simulink model "SimulateROSBag"  (R2020b)
settings: Solver=VariableStepAuto  StartTime=0.0  StopTime=80  RelTol=1e-3
PreLoadFcn:
  | load('turtleBotMazeMap.mat')
model workspace (MAT data in the model file):
  Logfile_Data_Object = robotics.ros.BagSelection
  Logfile_Data_Object.FilePath = 'C:\Users\josea\OneDrive - MathWorks\Desktop\RoboticsArena\Navigation_Series\MATLAB_Files\CreatingMaps\Data\ROSBag_turtleBotMaze.bag'
  Logfile_Data_Object.StartTime = 1574.403
  Logfile_Data_Object.EndTime = 1757.346
  Logfile_Data_Object.NumMessages = 6404
  Logfile_Data_Object.AvailableTopics = table
  Logfile_Data_Object.AvailableTopics.data{1} = [5489; 915]
  Logfile_Data_Object.AvailableTopics.data{2} = categorical
  Logfile_Data_Object.AvailableTopics.data{2}.categoryNames = {'nav_msgs/Odometry'; 'sensor_msgs/LaserScan'}
  Logfile_Data_Object.AvailableTopics.data{2}.codes = [1; 2]
  Logfile_Data_Object.AvailableTopics.data{3}{1} = '  uint32 Seq
    |   Time Stamp
    |   char FrameId
    | char ChildFrameId
    | geometry_msgs/PoseWithCovariance Pose
    |   geometry_msgs/Pose Pose
    |     geometry_msgs/Point Position
    |       double X
    |       double Y
    |       double Z
    |     geometry_msgs/Quaternion Orientation
    |       double X
    |       double Y
    |       double Z
    |       double W
    |   double[36] Covariance
    | geometry_msgs/TwistWithCovariance Twist
    |   geometry_msgs/Twist Twist
    |     geometry_msgs/Vector3 Linear
    |       double X
    |       double Y
    |       double Z
    |     geometry_msgs/Vector3 Angular
    |       double X
    |       double Y
    |       double Z
    |   double[36] Covariance
    | '
  Logfile_Data_Object.AvailableTopics.data{3}{2} = '  uint32 Seq
    |   Time Stamp
    |   char FrameId
    | single AngleMin
    | single AngleMax
    | single AngleIncrement
    | single TimeIncrement
    | single ScanTime
    | single RangeMin
    | single RangeMax
    | single[] Ranges
    | single[] Intensities
    | '
  Logfile_Data_Object.AvailableTopics.ndims = 2
  Logfile_Data_Object.AvailableTopics.nrows = 2
  Logfile_Data_Object.AvailableTopics.rownames = {'/odom'; '/scan'}
  Logfile_Data_Object.AvailableTopics.nvars = 3
  Logfile_Data_Object.AvailableTopics.varnames = {'NumMessages', 'MessageType', 'MessageDefinition'}
  Logfile_Data_Object.AvailableTopics.props.useVariableNamesOriginal = 0
  Logfile_Data_Object.AvailableTopics.props.useDimensionNamesOriginal = 0
  Logfile_Data_Object.AvailableTopics.props.CustomProps = struct()
  Logfile_Data_Object.AvailableTopics.props.VariableCustomProps = struct()
  Logfile_Data_Object.AvailableTopics.props.versionSavedFrom = 4
  Logfile_Data_Object.AvailableTopics.props.minCompatibleVersion = 1
  Logfile_Data_Object.AvailableTopics.props.incompatibilityMsg = ''
  Logfile_Data_Object.AvailableTopics.props.VersionSavedFrom = 4
  Logfile_Data_Object.AvailableTopics.props.Description = ''
  Logfile_Data_Object.AvailableTopics.props.VariableNamesOriginal = {}
  Logfile_Data_Object.AvailableTopics.props.DimensionNames = {'Row', 'Variables'}
  Logfile_Data_Object.AvailableTopics.props.DimensionNamesOriginal = {}
  Logfile_Data_Object.AvailableTopics.props.UserData = []
  Logfile_Data_Object.AvailableTopics.props.VariableDescriptions = {}
  Logfile_Data_Object.AvailableTopics.props.VariableUnits = {}
  Logfile_Data_Object.AvailableTopics.props.VariableContinuity = {}
  Logfile_Data_Object.MessageList = table
  Logfile_Data_Object.MessageList.data{1} = [1574.403 1574.437 1574.469 1574.502 1574.503 1574.537 1574.57 1574.603 1574.637 1574.67 1574.702 1574.704 ... (6404 elements, 6404x1)]
  Logfile_Data_Object.MessageList.data{2} = categorical
  Logfile_Data_Object.MessageList.data{2}.categoryNames = {'/odom'; '/scan'}
  Logfile_Data_Object.MessageList.data{2}.codes = [1 1 1 2 1 1 1 1 1 1 1 2 ... (6404 elements, 6404x1)]
  Logfile_Data_Object.MessageList.data{3} = categorical
  Logfile_Data_Object.MessageList.data{3}.categoryNames = {'nav_msgs/Odometry'; 'sensor_msgs/LaserScan'}
  Logfile_Data_Object.MessageList.data{3}.codes = [1 1 1 2 1 1 1 1 1 1 1 2 ... (6404 elements, 6404x1)]
  Logfile_Data_Object.MessageList.data{4} = [7630 8394 9158 12284 15271 16035 16799 17563 18327 19091 19855 20619 ... (6404 elements, 6404x1)]
  Logfile_Data_Object.MessageList.ndims = 2
  Logfile_Data_Object.MessageList.nrows = 6404
  Logfile_Data_Object.MessageList.nvars = 4
  Logfile_Data_Object.MessageList.varnames = {'Time', 'Topic', 'MessageType', 'FileOffset'}
  Logfile_Data_Object.MessageList.props.useVariableNamesOriginal = 0
  Logfile_Data_Object.MessageList.props.useDimensionNamesOriginal = 0
  Logfile_Data_Object.MessageList.props.CustomProps = struct()
  Logfile_Data_Object.MessageList.props.VariableCustomProps = struct()
  Logfile_Data_Object.MessageList.props.versionSavedFrom = 4
  Logfile_Data_Object.MessageList.props.minCompatibleVersion = 1
  Logfile_Data_Object.MessageList.props.incompatibilityMsg = ''
  Logfile_Data_Object.MessageList.props.VersionSavedFrom = 4
  Logfile_Data_Object.MessageList.props.Description = ''
  Logfile_Data_Object.MessageList.props.VariableNamesOriginal = {}
  Logfile_Data_Object.MessageList.props.DimensionNames = {'Row', 'Variables'}
  Logfile_Data_Object.MessageList.props.DimensionNamesOriginal = {}
  Logfile_Data_Object.MessageList.props.UserData = []
  Logfile_Data_Object.MessageList.props.VariableDescriptions = {}
  Logfile_Data_Object.MessageList.props.VariableUnits = {}
  Logfile_Data_Object.MessageList.props.VariableContinuity = {}
  Logfile_Data_Object.TopicTypeMap = containers.Map
  Logfile_Data_Object.TopicTypeMap.serialization.keys = {'/odom', '/scan'}
  Logfile_Data_Object.TopicTypeMap.serialization.values = {'nav_msgs/Odometry', 'sensor_msgs/LaserScan'}
  Logfile_Data_Object.TopicTypeMap.serialization.uniformity = 1
  Logfile_Data_Object.TopicTypeMap.serialization.keyType = 'char'
  Logfile_Data_Object.TopicTypeMap.serialization.valueType = 'char'
  Logfile_Data_Object.TopicDefinitionMap = containers.Map
  Logfile_Data_Object.TopicDefinitionMap.serialization.keys = {'/odom', '/scan'}
  Logfile_Data_Object.TopicDefinitionMap.serialization.values{1} = '  uint32 Seq
    |   Time Stamp
    |   char FrameId
    | char ChildFrameId
    | geometry_msgs/PoseWithCovariance Pose
    |   geometry_msgs/Pose Pose
    |     geometry_msgs/Point Position
    |       double X
    |       double Y
    |       double Z
    |     geometry_msgs/Quaternion Orientation
    |       double X
    |       double Y
    |       double Z
    |       double W
    |   double[36] Covariance
    | geometry_msgs/TwistWithCovariance Twist
    |   geometry_msgs/Twist Twist
    |     geometry_msgs/Vector3 Linear
    |       double X
    |       double Y
    |       double Z
    |     geometry_msgs/Vector3 Angular
    |       double X
    |       double Y
    |       double Z
    |   double[36] Covariance
    | '
  Logfile_Data_Object.TopicDefinitionMap.serialization.values{2} = '  uint32 Seq
    |   Time Stamp
    |   char FrameId
    | single AngleMin
    | single AngleMax
    | single AngleIncrement
    | single TimeIncrement
    | single ScanTime
    | single RangeMin
    | single RangeMax
    | single[] Ranges
    | single[] Intensities
    | '
  Logfile_Data_Object.TopicDefinitionMap.serialization.uniformity = 1
  Logfile_Data_Object.TopicDefinitionMap.serialization.keyType = 'char'
  Logfile_Data_Object.TopicDefinitionMap.serialization.valueType = 'char'
  Logfile_Data_Object.messageTypeMap = containers.Map
  Logfile_Data_Object.messageTypeMap.serialization.keys = {}
  Logfile_Data_Object.messageTypeMap.serialization.values = {}
  Logfile_Data_Object.messageTypeMap.serialization.uniformity = 0
  Logfile_Data_Object.messageTypeMap.serialization.keyType = 'char'
  Logfile_Data_Object.messageTypeMap.serialization.valueType = 'any'
  Logfile_Data_Object.Parser = robotics.ros.internal.tf.TransformationTreeParser
  Logfile_Path = 'C:\Users\josea\OneDrive - MathWorks\Desktop\RoboticsArena\Navigation_Series\MATLAB_Files\CreatingMaps\Data\ROSBag_turtleBotMaze.bag'
  Logfile_Playback_Duration = 80
  Logfile_Playback_Offset = 0
libraries: robotcorelib x1, robotlib x1, mobileRoboticsLib x1
settings Model: Creator=josea  LastModifiedBy=josea

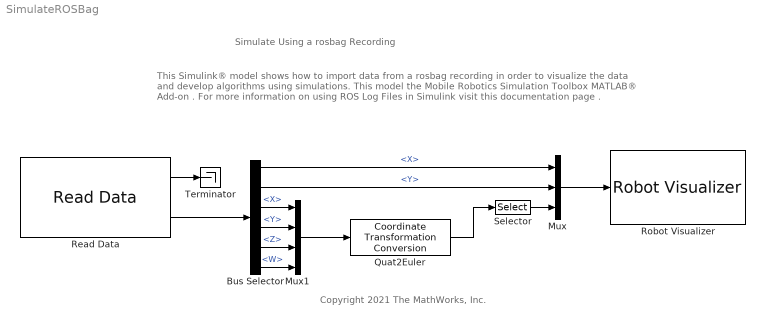
== system SimulateROSBag ==
  note: This Simulink® model shows how to import data from a rosbag recording in order to visualize the data and develop algorithms using simulations. This model the Mobile Robotics Simulation Toolbox MATLAB® Add-on . For more information on using ROS Log Files in Simulink visit this documentation page .
  note: Simulate Using a rosbag Recording
  note: Copyright 2021 The MathWorks, Inc.
  Bus Selector : BusSelector  OutputSignals=Pose.Pose.Position.X,Pose.Pose.Position.Y,Pose.Pose.Orientation.X,Pose.Pose.Orientation.Y,Pose.Pose.Orientation.Z,Pose.Pose.Orientation.W
  Mux : Mux  Inputs=3
  Mux1 : Mux
  Quat2Euler : robotcorelib/Coordinate Transformation Conversion  InputRepresentation=Quaternion  InputEulerSequence=ZYX  ShowTrVecInputPort=on  OutputRepresentation=Euler Angles  OutputEulerSequence=ZYX  ShowTrVecOutputPort=on  SimulateUsing=Interpreted execution
      settings: SourceProductBaseCode=NV,RO,RR,UV
  Read Data : robotlib/Read Data  topic=/odom  sampleTime=0.05  logfileType=rosbag  modelName=SimulateROSBag  msgType=nav_msgs/Odometry
      settings: SourceProductBaseCode=RR
  Robot Visualizer : mobileRoboticsLib/Environments/Robot Visualizer  robotRadius=0.2  mapName=myOccMap  showTrajectory=on  hasWaypoints=off  hasLidar=off  sensorOffset=[ 0, 0 ]  scanAngles=[ -pi/4, 0, pi/4 ]  hasObjDetector=off  objDetectorOffset=[ 0, 0 ]  objDetectorAngle=0  objDetectorFOV=pi/4  objDetectorMaxRange=5  objectColors=[ 1, 0, 0; 0, 1, 0; 0, 0, 1 ]  objectMarkers=s
  Selector : Selector  InputPortWidth=3  IndexOptions=Index vector (dialog)  Indices=3  OutputSizes=1
  Terminator : Terminator
  wires:
  Read Data/2 -> Bus Selector/1
  Bus Selector/1 -> Mux/1  "<X>"
  Bus Selector/2 -> Mux/2  "<Y>"
  Mux/1 -> Robot Visualizer/1
  Bus Selector/3 -> Mux1/1  "<X>"
  Bus Selector/4 -> Mux1/2  "<Y>"
  Bus Selector/5 -> Mux1/3  "<Z>"
  Bus Selector/6 -> Mux1/4  "<W>"
  Mux1/1 -> Quat2Euler/1
  Quat2Euler/1 -> Selector/1
  Selector/1 -> Mux/3
  Read Data/1 -> Terminator/1
